simulink model "KalmanWienerSimulation"  (R2019b)
settings: Solver=VariableStepAuto  StartTime=0.0  StopTime=10.0  RelTol=1e-3
values from neighbouring files (symbols this model uses):
  A_double = [0 1; 0 0]    [kalman_matrices_calculator.m]
  A_s_single = eval(subs(Ad_single,Ts))    [kalman_matrices_calculator.m]
  A_single = [0]    [kalman_matrices_calculator.m]
  B_double = [0; 1]    [kalman_matrices_calculator.m]
  B_s_single = eval(subs(Bd_single,Ts))    [kalman_matrices_calculator.m]
  B_single = [1]    [kalman_matrices_calculator.m]
  C_double = [1 0]    [kalman_matrices_calculator.m]
  C_single = [1]    [kalman_matrices_calculator.m]
  D_double = [0]    [kalman_matrices_calculator.m]
  D_single = [0]    [kalman_matrices_calculator.m]
  L_double = lqe(A_double, G_double, C_double, q_double, r_double, 0)    [kalman_matrices_calculator.m]
  L_single = lqe(A_single, G_single, C_single, q_single, r_single, 0)    [kalman_matrices_calculator.m]
  q_single = cov(out.In_Out_Data{1}.Values.Data)*10000000000000    [kalman_matrices_calculator.m]
  r_single = cov(out.In_Out_Data{2}.Values.Data)    [kalman_matrices_calculator.m]
  Ts = 0.005    [kalman_matrices_calculator.m]
undefined symbols (not defined in the file or in its folder): A_cont, A_s, B_cont, B_s, C_cont, D_cont, DiscIntNeverNeededParam, Discrete, L, q, r, Time
libraries: simulink x6, ctrlSharedLib x3
settings Model: Creator=Sankalp Bhan  LastModifiedBy=Chris

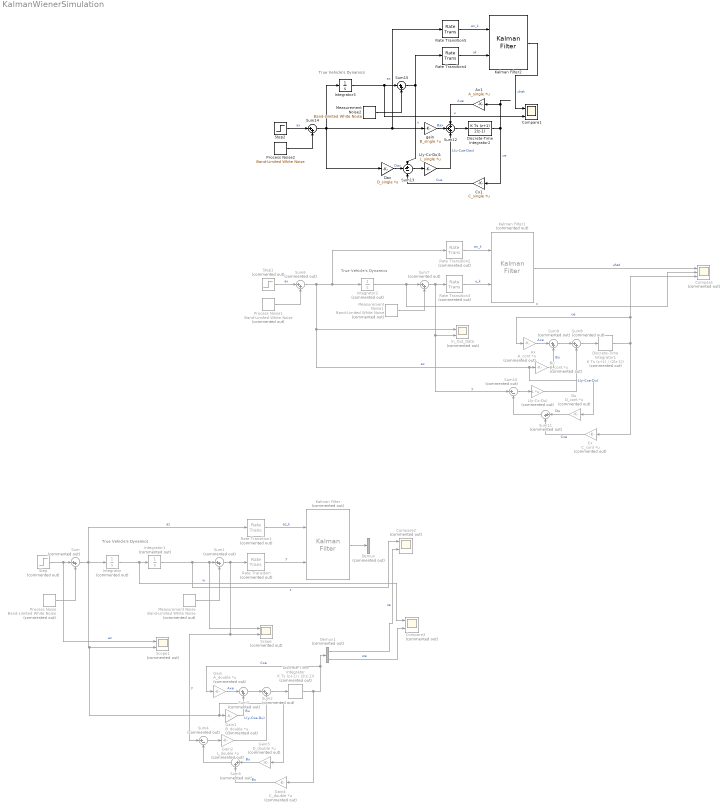
== system KalmanWienerSimulation ==
  note: True Vehicle's Dynamics
  note: True Vehicle's Dynamics
  note: True Vehicle's Dynamics
  Ax : Gain  Commented=on  Gain=A_cont  Multiplication=Matrix(K*u)
  Ax1 : Gain  Gain=A_single  Multiplication=Matrix(K*u)
      settings: AttributesFormatString=Ax
  Bu : Gain  Commented=on  Gain=B_cont  Multiplication=Matrix(K*u)
  Compare : Scope  Commented=on  NumInputPorts=3
  Compare1 : Scope  NumInputPorts=2
  Compare2 : Scope  Commented=on  NumInputPorts=2
  Compare3 : Scope  Commented=on  NumInputPorts=2
  Cx : Gain  Commented=on  Gain=C_cont  Multiplication=Matrix(K*u)
  Cx1 : Gain  Gain=C_single  Multiplication=Matrix(K*u)
      settings: AttributesFormatString=Cx
  Dax : Gain  Gain=D_single  Multiplication=Matrix(K*u)
      settings: AttributesFormatString=Du
  Demux : Demux  Commented=on  Outputs=2
  Demux1 : Demux  Commented=on  Outputs=2
  Discrete-Time Integrator : DiscreteIntegrator  Commented=on  IntegratorMethod=Integration: Trapezoidal  SampleTime=-1  ICPrevOutput=DiscIntNeverNeededParam  ICPrevScaledInput=DiscIntNeverNeededParam
  Discrete-Time Integrator1 : DiscreteIntegrator  Commented=on  IntegratorMethod=Integration: Trapezoidal  SampleTime=-1  ICPrevOutput=DiscIntNeverNeededParam  ICPrevScaledInput=DiscIntNeverNeededParam
  Discrete-Time Integrator2 : DiscreteIntegrator  IntegratorMethod=Integration: Trapezoidal  SampleTime=-1  ICPrevOutput=DiscIntNeverNeededParam  ICPrevScaledInput=DiscIntNeverNeededParam
  Du : Gain  Commented=on  Gain=D_cont  Multiplication=Matrix(K*u)
  Gain : Gain  Commented=on  Gain=A_double  Multiplication=Matrix(K*u)
  Gain1 : Gain  Commented=on  Gain=B_double  Multiplication=Matrix(K*u)
  Gain2 : Gain  Commented=on  Gain=L_double  Multiplication=Matrix(K*u)
  Gain3 : Gain  Commented=on  Gain=D_double  Multiplication=Matrix(K*u)
  Gain4 : Gain  Commented=on  Gain=C_double  Multiplication=Matrix(K*u)
  In_Out_Data : Scope  Commented=on  NumInputPorts=2
  Integrator : Integrator  Commented=on
  Integrator1 : Integrator  Commented=on
  Integrator2 : Integrator  Commented=on
  Integrator3 : Integrator
  Kalman Filter : ctrlSharedLib/Kalman Filter  Commented=on  TimeDomain=Discrete-Time  UseCurrentEstimator=on  ModelSource=Individual A, B, C, D matrices  ModelSourceVariable=ss(0.95,1,1,0,1)  A=[1 0.005 ; 0 1]  B="[0.005^2/2 ;  0.005]"  C=[1 0]  D=0  NumberOfStates=1  NumberOfInputs=1  NumberOfOutputs=1  InitialEstimateSource=Dialog  X0=[0;0 ]  P0=10  UseK=off  UseGH=off  NumberOfProcessNoiseInputs=1  G=1  TimeInvariantG=on  H=0  TimeInvariantH=on  Q=[0 0 ; 0 1]*q;  TimeInvariantQ=on  R=10*r;  TimeInvariantR=on  N=0  TimeInvariantN=on  AddInputPort=on  AddEnablePort=off  OutputEstimatedY=off  OutputP=off  Ts=-1
      settings: SourceProductBaseCode=CT
  Kalman Filter1 : ctrlSharedLib/Kalman Filter  Commented=on  TimeDomain=Discrete-Time  UseCurrentEstimator=on  ModelSource=Individual A, B, C, D matrices  ModelSourceVariable=ss(0.95,1,1,0,1)  A=A_s  B=B_s  C=[1]  D=0  NumberOfStates=1  NumberOfInputs=1  NumberOfOutputs=1  InitialEstimateSource=Dialog  X0=[0]  P0=10  UseK=off  UseGH=off  NumberOfProcessNoiseInputs=1  G=1  TimeInvariantG=on  H=0  TimeInvariantH=on  Q=[1]*q  TimeInvariantQ=on  R=[1]*r*10000  TimeInvariantR=on  N=0  TimeInvariantN=on  AddInputPort=on  AddEnablePort=off  OutputEstimatedY=off  OutputP=off  Ts=Ts
      settings: SourceProductBaseCode=CT
  Kalman Filter2 : ctrlSharedLib/Kalman Filter  TimeDomain=Discrete-Time  UseCurrentEstimator=on  ModelSource=Individual A, B, C, D matrices  ModelSourceVariable=ss(0.95,1,1,0,1)  A=A_s_single  B=B_s_single  C=C_single  D=D_single  NumberOfStates=1  NumberOfInputs=1  NumberOfOutputs=1  InitialEstimateSource=Dialog  X0=[0]  P0=10  UseK=off  UseGH=off  NumberOfProcessNoiseInputs=1  G=1  TimeInvariantG=on  H=0  TimeInvariantH=on  Q=[1]*q_single  TimeInvariantQ=on  R=[1]*r_single*10000  TimeInvariantR=on  N=0  TimeInvariantN=on  AddInputPort=on  AddEnablePort=off  OutputEstimatedY=off  OutputP=off  Ts=Ts
      settings: SourceProductBaseCode=CT
  L(y-Cx-Du) : Gain  Commented=on  Gain=L  Multiplication=Matrix(K*u)
  L(y-Cx-Du)1 : Gain  Gain=L_single  Multiplication=Matrix(K*u)
      settings: AttributesFormatString=L(y-Cx-Du)
  Measurement Noise : simulink/Sources/Band-Limited White Noise  Commented=on  Cov=[0.1]  Ts=0.005  seed=[23341]
  Measurement Noise1 : simulink/Sources/Band-Limited White Noise  Commented=on  Cov=[0.1]  Ts=0.005  seed=[23341]
  Measurement Noise2 : simulink/Sources/Band-Limited White Noise  Cov=[0.1]  Ts=0.005  seed=[23341]
  Process Noise : simulink/Sources/Band-Limited White Noise  Commented=on  Cov=[0.1]  Ts=0.005  seed=[23342]
  Process Noise1 : simulink/Sources/Band-Limited White Noise  Commented=on  Cov=[0.1]  Ts=0.005  seed=[23342]
  Process Noise2 : simulink/Sources/Band-Limited White Noise  Cov=[0.1]  Ts=0.005  seed=[23342]
  Rate Transition{,1..3} (4 alike) : RateTransition  Commented=on  OutPortSampleTime=0.005
  Rate Transition4 : RateTransition  OutPortSampleTime=0.005
  Rate Transition5 : RateTransition  OutPortSampleTime=0.005
  Scope : Scope  Commented=on  NumInputPorts=2
  Scope1 : Scope  Commented=on  NumInputPorts=2
  Step : Step  Commented=on  SampleTime=0
  Step1 : Step  Commented=on  SampleTime=0
  Step2 : Step  SampleTime=0
  Sum{,1..3,5..9,11} (10 alike) : Sum  Commented=on  Inputs=|++
  Sum10 : Sum  Commented=on  Inputs=|+-
  Sum12 : Sum  Inputs=+++
  Sum13 : Sum  Inputs=+--
  Sum14 : Sum  Inputs=|++
  Sum15 : Sum  Inputs=|++
  Sum4 : Sum  Commented=on  Inputs=|+-
  gain : Gain  Gain=B_single  Multiplication=Matrix(K*u)
      settings: AttributesFormatString=Bu
  wires:
  Integrator/1 -> Compare3/1, Integrator1/1  "w"
  Rate Transition/1 -> Kalman Filter/2  "y"
  Step/1 -> Scope1/1, Sum/1  "az"
  Process Noise/1 -> Sum/2
  Measurement Noise/1 -> Sum1/2
  Integrator1/1 -> Compare2/1, Scope/1, Sum1/1  "z"
  Rate Transition1/1 -> Kalman Filter/1  "az_k"
  Kalman Filter/1 -> Demux/1
  Demux1/2 -> Compare3/2  "we"
  Demux1/1 -> Compare2/2  "ze"
  Gain2/1 -> Sum2/2  "L(y-Cxe-Du)"
  Sum5/1 -> Sum4/2
  Sum3/1 -> Sum2/1
  Gain4/1 -> Sum5/2  "Bu"
  Gain/1 -> Sum3/1  "Axe"
  Sum2/1 -> Discrete-Time Integrator/1
  Sum4/1 -> Gain2/1
  Gain3/1 -> Sum5/1  "Bu"
  Discrete-Time Integrator/1 -> Gain4/1, Gain/1, Demux1/1  "Cxe"
  Gain1/1 -> Sum3/2  "Bu"
  Sum/1 -> Integrator/1, Rate Transition1/1, Gain1/1, Gain3/1, Scope1/2  "az"
  Sum1/1 -> Scope/2, Sum4/1, Rate Transition/1  "y"
  Step1/1 -> Sum6/1  "ax"
  Process Noise1/1 -> Sum6/2
  Integrator2/1 -> Compare/2, Sum7/1  "u"
  Measurement Noise1/1 -> Sum7/2
  Rate Transition2/1 -> Kalman Filter1/1  "ax_k"
  Rate Transition3/1 -> Kalman Filter1/2  "u_k"
  Kalman Filter1/1 -> Compare/1  "uhat"
  Sum7/1 -> Sum10/1, In_Out_Data/2, Rate Transition3/1  "y"
  Sum6/1 -> Du/1, Bu/1, In_Out_Data/1, Rate Transition2/1, Integrator2/1  "ax"
  Bu/1 -> Sum9/2  "Bu"
  Discrete-Time Integrator1/1 -> Compare/3, Ax/1, Cx/1  "ue"
  Du/1 -> Sum11/1  "Du"
  Sum10/1 -> L(y-Cx-Du)/1
  Sum8/1 -> Discrete-Time Integrator1/1
  Ax/1 -> Sum9/1  "Axe"
  Cx/1 -> Sum11/2  "Cxe"
  Sum9/1 -> Sum8/1
  Sum11/1 -> Sum10/2
  L(y-Cx-Du)/1 -> Sum8/2  "L(y-Cxe-Du)"
  Dax/1 -> Sum13/2  "Dax"
  Ax1/1 -> Sum12/1  "Aue"
  Discrete-Time Integrator2/1 -> Ax1/1, Cx1/1  "ue"
  Sum13/1 -> L(y-Cx-Du)1/1
  Cx1/1 -> Sum13/3  "Cue"
  gain/1 -> Sum12/2  "Bax"
  Sum12/1 -> Discrete-Time Integrator2/1
  L(y-Cx-Du)1/1 -> Sum12/3  "L(u-Cue-Dax)"
  Process Noise2/1 -> Sum14/2
  Step2/1 -> Sum14/1  "ax"
  Measurement Noise2/1 -> Sum15/2
  Integrator3/1 -> Compare1/2, Sum15/1  "u"
  Sum15/1 -> Rate Transition4/1, Sum13/1  "u"
  Kalman Filter2/1 -> Compare1/1  "uhat"
  Sum14/1 -> Rate Transition5/1, gain/1, Integrator3/1, Dax/1  "ax"
  Rate Transition4/1 -> Kalman Filter2/2  "uk"
  Rate Transition5/1 -> Kalman Filter2/1  "ax_k"
